simulink model "Sem1DemoSmallANDTOU_COPY"  (R2023a)
settings: Solver=ode23t  StartTime=0.0  StopTime=10  RelTol=1e-3
libraries: simulink x15, dspswit3 x9, simulink_extras x7, spspowerguiLib x1
settings Model: PacingRate=4  Creator=jakob  LastModifiedBy=matty

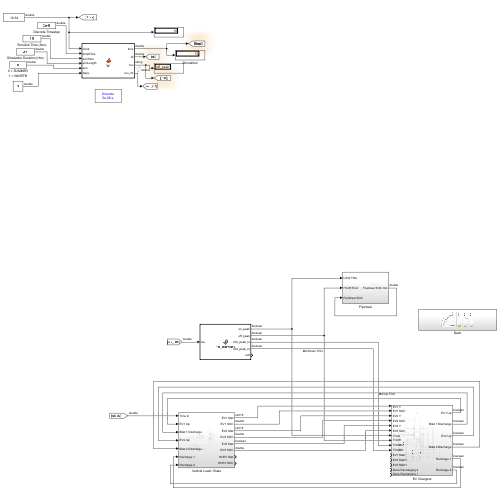
[thumbnail: Simulink's stored preview of the top-level diagram]
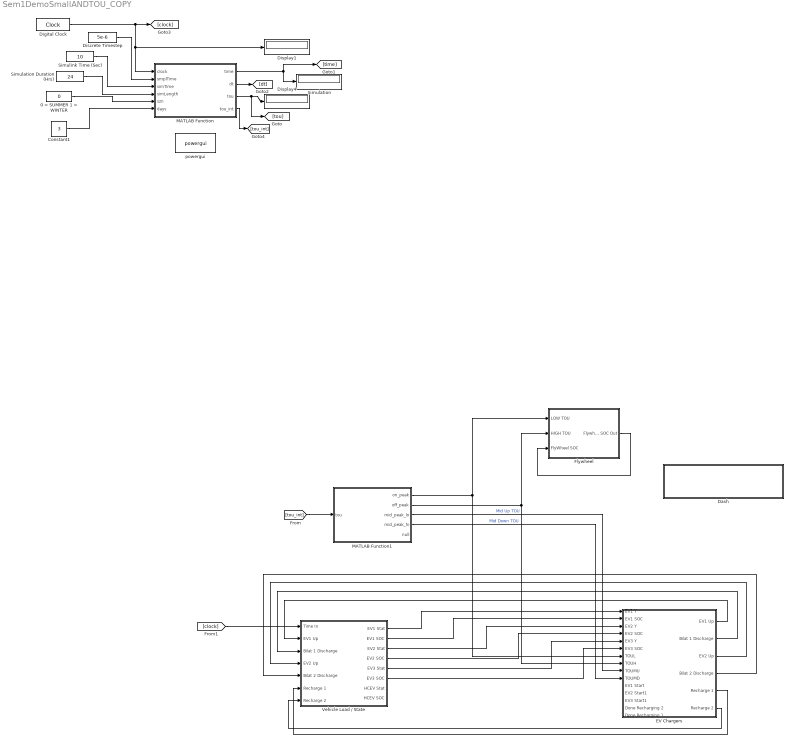
== system Sem1DemoSmallANDTOU_COPY ==
  0 = SUMMER 1 = WINTER : Constant  Value=0
  Constant1 : Constant  Value=3
  Dash : Subsystem
  Digital Clock : DigitalClock  SampleTime=5e-6
  Discrete Timestep : Constant  Value=5e-6
  Display1 : Display
  Display4 : Display
  EV Chargers : Subsystem
  Flywheel : Subsystem  StopFcn=CapTest
  MATLAB Function : MATLAB Function  TreatAsAtomicUnit=on
  MATLAB Function1 : MATLAB Function  TreatAsAtomicUnit=on
  Simulation : Display
  Simulation Duration (Hrs) : Constant  Value=24
  Simulink Time (Sec) : Constant  Value=10
  Vehicle Load / State : Subsystem
  powergui : spspowerguiLib/powergui  Priority=1  SimulationMode=Discrete  SampleTime=5e-6  frequency=60  Iterations=50  frequencyindice=0  Pbase=100e6  ErrMax=1e-4  UnitsV=kV  UnitsW=MW  buscounter=0  FunctionMessages=off  echomessages=off  EnableUseOfTLC=off  CurrentSourceSwitches=off  DisableSnubberDevices=off  DisableRonSwitches=off  DisableVfSwitches=off  DisplayEquations=off  AutomaticDiscreteSolvers=off  SolverType=Tustin/Backward Euler (TBE)  Interpol=off  ExternalGateDelay=off  methode=off  Ts=100  x0status=blocks  SPID=on  SwTol=0  HookPort=off  NonlinearTolerance=1e-4  nMaxIteration=100  ContinueOnMaxIteration=off  RestoreLinks=warning  ResistiveCurrentMeasurement=off  Frange=[0:2:500]  Ylog=off  Xlog=on  ShowGrid=off  save=off  variable=ZData  structure=0  ZoomFFT=off  StartTime=0.0  cycles=1  DisplayStyle=1  fundamental=60  FreqAxis=off  MaxFrequency=1000  frequencyindicesteady=1  RmsSteady=1  display=off
  wires:
  MATLAB Function1/1(on_peak) -> EV Chargers/7(TOUL), Flywheel/1(LOW TOU)
  Vehicle Load / State/1(EV1 Stat) -> EV Chargers/1(EV1 Y)
  Vehicle Load / State/2(EV1 SOC) -> EV Chargers/2(EV1 SOC)
  Vehicle Load / State/3(EV2 Stat) -> EV Chargers/3(EV2 Y)
  Vehicle Load / State/4(EV2 SOC) -> EV Chargers/4(EV2 SOC)
  Vehicle Load / State/5(EV3 Stat) -> EV Chargers/5(EV3 Y)
  Vehicle Load / State/6(EV3 SOC) -> EV Chargers/6(EV3 SOC)
  MATLAB Function1/2(off_peak) -> EV Chargers/8(TOUH), Flywheel/2(HIGH TOU)
  MATLAB Function1/3(mid_peak_lo) -> EV Chargers/9(TOUMU)  "Mid Up TOU"
  MATLAB Function1/4(mid_peak_hi) -> EV Chargers/10(TOUMD)  "Mid Down TOU"
  Flywheel/1(Flywheel SOC Out) -> Flywheel/3(FlyWheel SOC)
  EV Chargers/1(EV1 Up) -> Vehicle Load / State/2(EV1 Up)
  EV Chargers/2(Bilat 1 Discharge) -> Vehicle Load / State/3(Bilat 1 Discharge)
  EV Chargers/3(EV2 Up) -> Vehicle Load / State/4(EV2 Up)
  EV Chargers/4(Bilat 2 Discharge) -> Vehicle Load / State/5(Bilat 2 Discharge)
  EV Chargers/5(Recharge 1) -> Vehicle Load / State/6(Recharge 1)
  EV Chargers/6(Recharge 2) -> Vehicle Load / State/7(Recharge 2)
  MATLAB Function/4(tou_int) -> [tou_int]
  0 = SUMMER 1 = WINTER/1 -> MATLAB Function/5(szn)
  Constant1/1 -> MATLAB Function/6(days)
  MATLAB Function/2(dt) -> [dt]
  Simulink Time (Sec)/1 -> MATLAB Function/3(simTime)
  MATLAB Function/3(tou) -> [tou], Display4/1
  Discrete Timestep/1 -> MATLAB Function/2(smplTime)
  Digital Clock/1 -> [clock], MATLAB Function/1(clock), Display1/1
  MATLAB Function/1(time) -> [time], Simulation/1
  Simulation Duration (Hrs)/1 -> MATLAB Function/4(simLength)
  [tou_int] -> MATLAB Function1/1(tou)
  [clock] -> Vehicle Load / State/1(Time In)

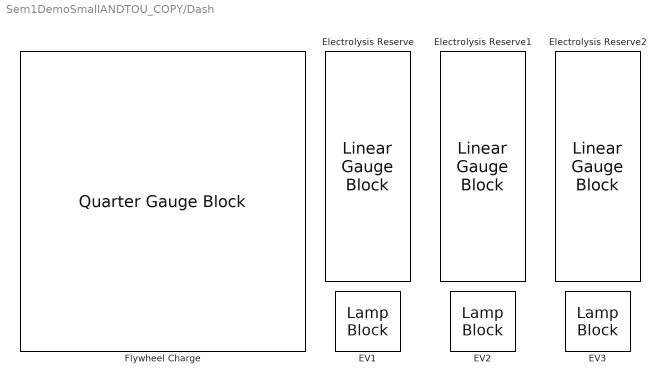
== system Sem1DemoSmallANDTOU_COPY/Dash ==
  EV1 : LampBlock  LabelPosition=Hide
  EV2 : LampBlock  LabelPosition=Hide
  EV3 : LampBlock  LabelPosition=Hide
  Electrolysis Reserve : LinearGaugeBlock  Tag=Flywheel %
  Electrolysis Reserve1 : LinearGaugeBlock  Tag=Flywheel %
  Electrolysis Reserve2 : LinearGaugeBlock  Tag=Flywheel %
  Flywheel Charge : QuarterGaugeBlock

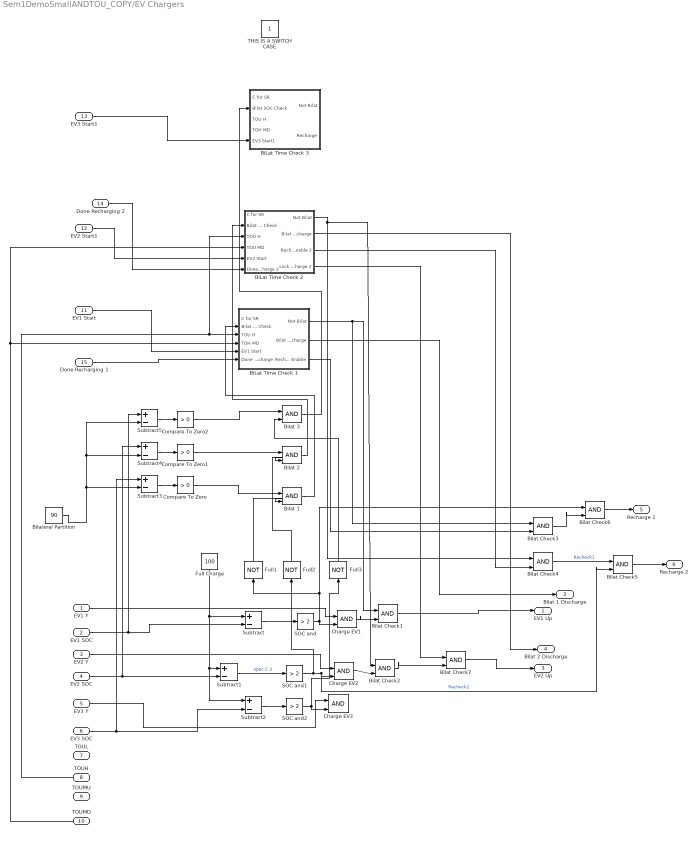
== system Sem1DemoSmallANDTOU_COPY/EV Chargers ==
  EV1 Y : Inport
  EV1 SOC : Inport  Port=2
  EV2 Y : Inport  Port=3
  EV2 SOC : Inport  Port=4
  EV3 Y : Inport  Port=5
  EV3 SOC : Inport  Port=6
  TOUL : Inport  Port=7
  TOUH : Inport  Port=8
  TOUMU : Inport  Port=9
  TOUMD : Inport  Port=10
  EV1 Start : Inport  Port=11
  EV2 Start1 : Inport  Port=12
  EV3 Start1 : Inport  Port=13
  Done Recharging 2 : Inport  Port=14
  Done Recharging 1 : Inport  Port=15
  BiLat Time Check 1 : Subsystem
  BiLat Time Check 2 : Subsystem
  BiLat Time Check 3 : Subsystem
  Bilat 1 : Logic  IconShape=distinctive  AllPortsSameDT=off  OutDataTypeStr=boolean
  Bilat 2 : Logic  IconShape=distinctive  AllPortsSameDT=off  OutDataTypeStr=boolean
  Bilat 3 : Logic  IconShape=distinctive  AllPortsSameDT=off  OutDataTypeStr=boolean
  Bilat Check{1..7} (7 alike) : Logic  IconShape=distinctive  AllPortsSameDT=off  OutDataTypeStr=boolean
  Bilateral Partition : Constant  Value=90
  Charge EV1 : Logic  IconShape=distinctive  AllPortsSameDT=off  OutDataTypeStr=boolean
  Charge EV2 : Logic  IconShape=distinctive  AllPortsSameDT=off  OutDataTypeStr=boolean
  Charge EV3 : Logic  IconShape=distinctive  AllPortsSameDT=off  OutDataTypeStr=boolean
  Compare To Zero : simulink/Logic and Bit Operations/Compare To Zero  relop=>  OutDataTypeStr=boolean
  Compare To Zero1 : simulink/Logic and Bit Operations/Compare To Zero  relop=>  OutDataTypeStr=boolean
  Compare To Zero2 : simulink/Logic and Bit Operations/Compare To Zero  relop=>  OutDataTypeStr=boolean
  Full Charge : Constant  Value=100
  Full1 : Logic  Operator=NOT  IconShape=distinctive  AllPortsSameDT=off  OutDataTypeStr=boolean
  Full2 : Logic  Operator=NOT  IconShape=distinctive  AllPortsSameDT=off  OutDataTypeStr=boolean
  Full3 : Logic  Operator=NOT  IconShape=distinctive  AllPortsSameDT=off  OutDataTypeStr=boolean
  SOC and : simulink/Logic and Bit Operations/Compare To Constant  relop=>  const=2  OutDataTypeStr=boolean
  SOC and1 : simulink/Logic and Bit Operations/Compare To Constant  relop=>  const=2  OutDataTypeStr=boolean
  SOC and2 : simulink/Logic and Bit Operations/Compare To Constant  relop=>  const=2  OutDataTypeStr=boolean
  Subtract{,1..5} (6 alike) : Sum  Inputs=+-
  THIS IS A SWITCH CASE : Constant
  EV1 Up : Outport
  Bilat 1 Discharge : Outport  Port=2
  EV2 Up : Outport  Port=3
  Bilat 2 Discharge : Outport  Port=4
  Recharge 1 : Outport  Port=5
  Recharge 2 : Outport  Port=6
  wires:
  Full Charge/1 -> Subtract2/1, Subtract1/1, Subtract/1
  EV1 SOC/1 -> Subtract5/1, Subtract/2
  EV2 Y/1 -> Charge EV2/1
  SOC and1/1 -> Bilat Check5/2, Charge EV2/2, Full2/1  "Recheck2"
  Subtract1/1 -> SOC and1/1  "Spec C 3"
  SOC and2/1 -> Full3/1, Charge EV3/2
  SOC and/1 -> Bilat Check6/1, Full1/1, Charge EV1/2
  Subtract/1 -> SOC and/1
  Subtract2/1 -> SOC and2/1
  EV3 SOC/1 -> Subtract3/1, Subtract2/2
  Charge EV2/1 -> Bilat Check2/2
  EV1 Y/1 -> Charge EV1/1
  EV3 Y/1 -> Charge EV3/1
  EV2 SOC/1 -> Subtract4/1, Subtract1/2
  Subtract3/1 -> Compare To Zero/1
  Subtract4/1 -> Compare To Zero1/1
  Subtract5/1 -> Compare To Zero2/1
  Full1/1 -> Bilat 1/2
  Compare To Zero/1 -> Bilat 1/1
  Compare To Zero1/1 -> Bilat 2/1
  Compare To Zero2/1 -> Bilat 3/1
  Full2/1 -> Bilat 2/2
  Full3/1 -> Bilat 3/2
  Bilateral Partition/1 -> Subtract4/2, Subtract5/2, Subtract3/2
  Bilat 3/1 -> BiLat Time Check 3/2(Bilat SOC Check)
  Bilat 2/1 -> BiLat Time Check 2/2(Bilat SOC Check)
  EV1 Start/1 -> BiLat Time Check 1/5(EV1 Start)
  Bilat 1/1 -> BiLat Time Check 1/2(Bilat SOC Check)
  TOUH/1 -> BiLat Time Check 2/3(TOU H), BiLat Time Check 1/3(TOU H)
  TOUMD/1 -> BiLat Time Check 2/4(TOU MD), BiLat Time Check 1/4(TOH MD)
  BiLat Time Check 1/2(Bilat Discharge) -> Bilat 1 Discharge/1
  BiLat Time Check 1/1(Not Bilat) -> Bilat Check3/1, Bilat Check1/1
  Charge EV1/1 -> Bilat Check1/2
  EV2 Start1/1 -> BiLat Time Check 2/5(EV2 Start)
  EV3 Start1/1 -> BiLat Time Check 3/5(EV3 Start1)
  BiLat Time Check 2/1(Not Bilat) -> Bilat Check4/1, Bilat Check2/1
  BiLat Time Check 2/2(Bilat Discharge) -> Bilat 2 Discharge/1
  Bilat Check2/1 -> Bilat Check7/2
  Bilat Check1/1 -> EV1 Up/1
  BiLat Time Check 1/3(Recharge Enable) -> Bilat Check3/2
  BiLat Time Check 2/3(Recharge Enable 2) -> Bilat Check4/2
  Done Recharging 2/1 -> BiLat Time Check 2/6(Done Recharge 2)
  Done Recharging 1/1 -> BiLat Time Check 1/6(Done Recharge)
  Bilat Check3/1 -> Bilat Check6/2
  Bilat Check4/1 -> Bilat Check5/1  "Recheck1"
  Bilat Check5/1 -> Recharge 2/1
  Bilat Check6/1 -> Recharge 1/1
  Bilat Check7/1 -> EV2 Up/1
  BiLat Time Check 2/4(Lock Out Recharge 2) -> Bilat Check7/1

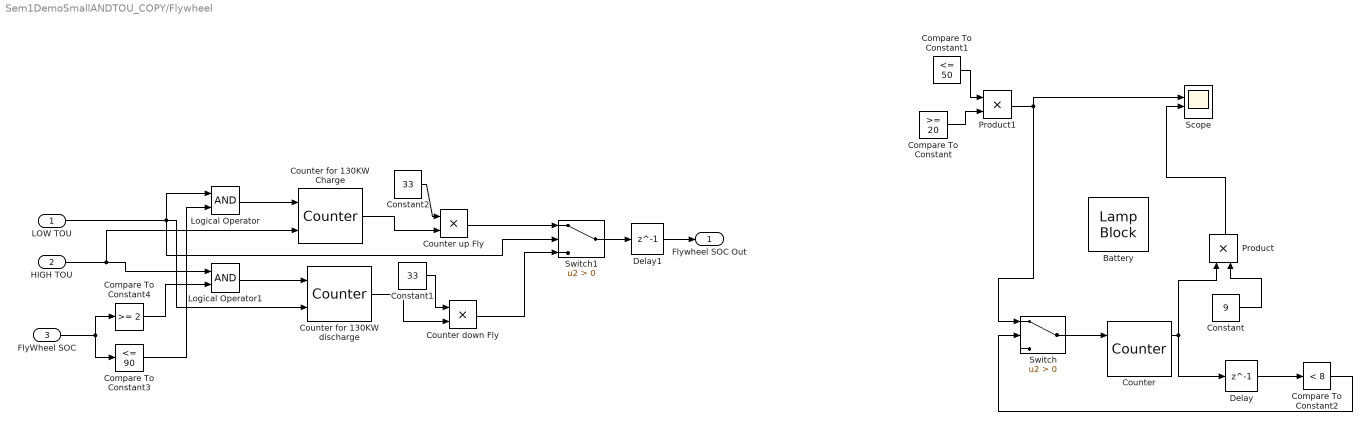
== system Sem1DemoSmallANDTOU_COPY/Flywheel ==
  LOW TOU : Inport
  HIGH TOU : Inport  Port=2
  FlyWheel SOC : Inport  Port=3
  Battery : LampBlock  LabelPosition=Hide  Icon=Battery
  Compare To Constant : simulink/Logic and Bit Operations/Compare To Constant  relop=>=  const=20  OutDataTypeStr=boolean
  Compare To Constant1 : simulink/Logic and Bit Operations/Compare To Constant  relop=<=  const=50  OutDataTypeStr=boolean
  Compare To Constant2 : simulink/Logic and Bit Operations/Compare To Constant  relop=<  const=8  OutDataTypeStr=boolean
  Compare To Constant3 : simulink/Logic and Bit Operations/Compare To Constant  relop=<=  const=90  OutDataTypeStr=boolean
  Compare To Constant4 : simulink/Logic and Bit Operations/Compare To Constant  relop=>=  const=2  OutDataTypeStr=boolean
  Constant : Constant  Value=9
  Constant1 : Constant  Value=33
  Constant2 : Constant  Value=33
  Counter : dspswit3/Counter  Direction=Up  CountEvent=Non-zero sample  CounterSize=User defined  MaxCount=100  InitialCount=0  Output=Count and Hit  HitValue=32  ResetInput=on  SamplesPerFrame=1  Ts=1  CntDtype=single  HitDtype=Logical
  Counter down Fly : Product
  Counter for 130KW Charge : dspswit3/Counter  Direction=Up  CountEvent=Non-zero sample  CounterSize=User defined  MaxCount=3  InitialCount=0  Output=Count  HitValue=32  ResetInput=on  SamplesPerFrame=1  Ts=1  CntDtype=single  HitDtype=Logical
  Counter for 130KW discharge : dspswit3/Counter  Direction=Down  CountEvent=Non-zero sample  CounterSize=User defined  MaxCount=10  InitialCount=3  Output=Count  HitValue=32  ResetInput=on  SamplesPerFrame=1  Ts=1  CntDtype=single  HitDtype=Logical
  Counter up Fly : Product
  Delay : Delay  DelayLength=1  InitialCondition=0
  Delay1 : Delay  DelayLength=1  InitialCondition=0
  Logical Operator : Logic  AllPortsSameDT=off  OutDataTypeStr=boolean
  Logical Operator1 : Logic  AllPortsSameDT=off  OutDataTypeStr=boolean
  Product : Product
  Product1 : Product
  Scope : Scope  NumInputPorts=4
  Switch : Switch  Criteria=u2 > Threshold  SaturateOnIntegerOverflow=off  InputSameDT=off
  Switch1 : Switch  Criteria=u2 > Threshold  SaturateOnIntegerOverflow=off  InputSameDT=off
  Flywheel SOC Out : Outport
  wires:
  Compare To Constant1/1 -> Product1/1
  Compare To Constant/1 -> Product1/2
  Counter/1 -> Product/1, Delay/1
  Product1/1 -> Switch/1, Scope/2
  Switch/1 -> Counter/1
  Compare To Constant2/1 -> Switch/2
  Delay/1 -> Compare To Constant2/1
  Constant/1 -> Product/2
  Product/1 -> Scope/3
  LOW TOU/1 -> Counter for 130KW discharge/2, Logical Operator/1, Switch1/2
  FlyWheel SOC/1 -> Compare To Constant4/1, Compare To Constant3/1
  Compare To Constant3/1 -> Logical Operator/2
  Compare To Constant4/1 -> Logical Operator1/2
  HIGH TOU/1 -> Counter for 130KW Charge/2, Logical Operator1/1
  Logical Operator1/1 -> Counter for 130KW discharge/1
  Constant1/1 -> Counter down Fly/1
  Counter for 130KW discharge/1 -> Counter down Fly/2
  Counter down Fly/1 -> Switch1/3
  Constant2/1 -> Counter up Fly/1
  Counter for 130KW Charge/1 -> Counter up Fly/2
  Logical Operator/1 -> Counter for 130KW Charge/1
  Counter up Fly/1 -> Switch1/1
  Switch1/1 -> Delay1/1
  Delay1/1 -> Flywheel SOC Out/1

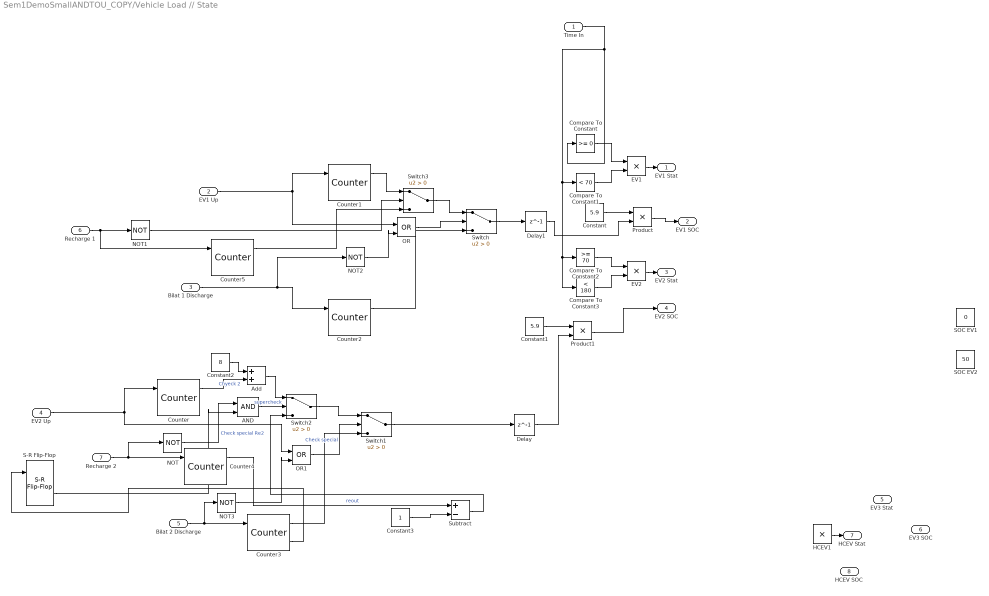
== system Sem1DemoSmallANDTOU_COPY/Vehicle Load // State ==
  Time In : Inport
  EV1 Up : Inport  Port=2
  Bilat 1 Discharge : Inport  Port=3
  EV2 Up : Inport  Port=4
  Bilat 2 Discharge : Inport  Port=5
  Recharge 1 : Inport  Port=6
  Recharge 2 : Inport  Port=7
  AND : Logic  IconShape=distinctive  AllPortsSameDT=off  OutDataTypeStr=boolean
  Add : Sum
  Compare To Constant : simulink/Logic and Bit Operations/Compare To Constant  relop=>=  const=0  OutDataTypeStr=boolean
  Compare To Constant1 : simulink/Logic and Bit Operations/Compare To Constant  relop=<  const=70  OutDataTypeStr=boolean
  Compare To Constant2 : simulink/Logic and Bit Operations/Compare To Constant  relop=>=  const=70  OutDataTypeStr=boolean
  Compare To Constant3 : simulink/Logic and Bit Operations/Compare To Constant  relop=<  const=180  OutDataTypeStr=boolean
  Constant : Constant  Value=5.9
  Constant1 : Constant  Value=5.9
  Constant2 : Constant  Value=8
  Constant3 : Constant
  Counter : dspswit3/Counter  Direction=Up  CountEvent=Non-zero sample  CounterSize=User defined  MaxCount=17  InitialCount=0  Output=Count and Hit  HitValue=9  ResetInput=on  SamplesPerFrame=1  Ts=1  CntDtype=single  HitDtype=Logical
  Counter1 : dspswit3/Counter  Direction=Up  CountEvent=Non-zero sample  CounterSize=User defined  MaxCount=100  InitialCount=0  Output=Count and Hit  HitValue=32  ResetInput=on  SamplesPerFrame=1  Ts=1  CntDtype=single  HitDtype=Logical
  Counter2 : dspswit3/Counter  Direction=Down  CountEvent=Non-zero sample  CounterSize=User defined  MaxCount=100  InitialCount=17  Output=Count and Hit  HitValue=32  ResetInput=on  SamplesPerFrame=1  Ts=1  CntDtype=single  HitDtype=Logical
  Counter3 : dspswit3/Counter  Direction=Down  CountEvent=Non-zero sample  CounterSize=User defined  MaxCount=17  InitialCount=17  Output=Count and Hit  HitValue=15  ResetInput=on  SamplesPerFrame=1  Ts=1  CntDtype=single  HitDtype=Logical
  Counter4 : dspswit3/Counter  Direction=Up  CountEvent=Non-zero sample  CounterSize=User defined  MaxCount=18  InitialCount=15  Output=Count and Hit  HitValue=100  ResetInput=on  SamplesPerFrame=1  Ts=1  CntDtype=single  HitDtype=Logical
  Counter5 : dspswit3/Counter  Direction=Up  CountEvent=Non-zero sample  CounterSize=User defined  MaxCount=100  InitialCount=15  Output=Count and Hit  HitValue=32  ResetInput=on  SamplesPerFrame=1  Ts=1  CntDtype=single  HitDtype=Logical
  Delay : Delay  DelayLength=1  InitialCondition=0
  Delay1 : Delay  DelayLength=1  InitialCondition=0
  EV1 : Product
  EV2 : Product
  HCEV1 : Product
  NOT{,1..3} (4 alike) : Logic  Operator=NOT  IconShape=distinctive  AllPortsSameDT=off  OutDataTypeStr=boolean
  OR : Logic  Operator=OR  IconShape=distinctive  AllPortsSameDT=off  OutDataTypeStr=boolean
  OR1 : Logic  Operator=OR  IconShape=distinctive  AllPortsSameDT=off  OutDataTypeStr=boolean
  Product : Product
  Product1 : Product
  S-R Flip-Flop : simulink_extras/Flip Flops/S-R Flip-Flop  initial_condition=0
  SOC EV1 : Constant  Value=0
  SOC EV2 : Constant  Value=50
  Subtract : Sum  Inputs=+-
  Switch{,1..3} (4 alike) : Switch  Criteria=u2 > Threshold  SaturateOnIntegerOverflow=off  InputSameDT=off
  EV1 Stat : Outport
  EV1 SOC : Outport  Port=2
  EV2 Stat : Outport  Port=3
  EV2 SOC : Outport  Port=4
  EV3 Stat : Outport  Port=5
  EV3 SOC : Outport  Port=6
  HCEV Stat : Outport  Port=7
  HCEV SOC : Outport  Port=8
  wires:
  Time In/1 -> Compare To Constant3/1, Compare To Constant2/1, Compare To Constant1/1, Compare To Constant/1
  Compare To Constant3/1 -> EV2/2
  Compare To Constant2/1 -> EV2/1
  Compare To Constant/1 -> EV1/1
  Compare To Constant1/1 -> EV1/2
  EV2/1 -> EV2 Stat/1
  HCEV1/1 -> HCEV Stat/1
  EV1/1 -> EV1 Stat/1
  EV2 Up/1 -> OR1/1, Counter/1
  EV1 Up/1 -> OR/1, Counter1/1
  Bilat 1 Discharge/1 -> NOT2/1, Counter2/1
  Switch/1 -> Delay1/1
  Counter2/1 -> Switch/3
  Switch1/1 -> Delay/1
  Bilat 2 Discharge/1 -> NOT3/1, Counter3/1
  Switch2/1 -> Switch1/1
  Counter/1 -> Add/2  "Chyeck 2"
  Recharge 2/1 -> NOT/1, Counter4/1
  NOT/1 -> AND/1  "Check special Re2"
  Counter5/1 -> Switch3/3
  Recharge 1/1 -> Counter5/1, NOT1/1
  Counter1/1 -> Switch3/1
  Switch3/1 -> Switch/1
  NOT1/1 -> Switch3/2
  Delay/1 -> Product1/2
  Delay1/1 -> Product/2
  Constant/1 -> Product/1
  Product/1 -> EV1 SOC/1
  OR/1 -> Switch/2
  NOT2/1 -> OR/2
  NOT3/1 -> OR1/2
  OR1/1 -> Switch1/2  "Check special"
  Constant1/1 -> Product1/1
  Product1/1 -> EV2 SOC/1
  Constant2/1 -> Add/1
  Add/1 -> Switch2/1
  Counter3/2 -> S-R Flip-Flop/1
  S-R Flip-Flop/2 -> AND/2
  AND/1 -> Switch2/2  "supercheck"
  Counter3/1 -> Switch1/3
  Counter4/1 -> Subtract/1  "reout"
  Constant3/1 -> Subtract/2
  Subtract/1 -> Switch2/3

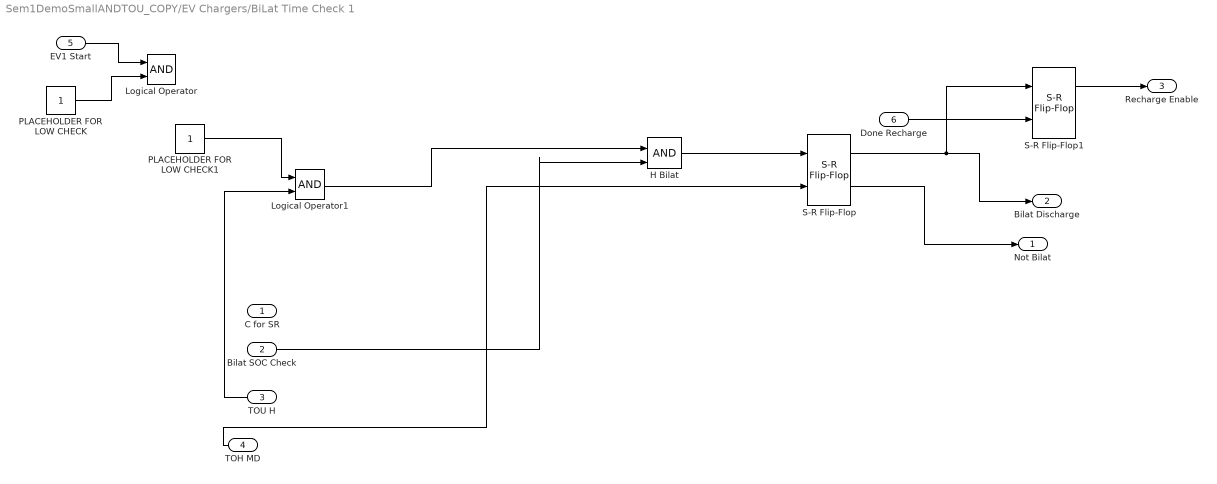
== system Sem1DemoSmallANDTOU_COPY/EV Chargers/BiLat Time Check 1 ==
  C for SR : Inport
  Bilat SOC Check : Inport  Port=2
  TOU H : Inport  Port=3
  TOH MD : Inport  Port=4
  EV1 Start : Inport  Port=5
  Done Recharge : Inport  Port=6
  H Bilat : Logic  IconShape=distinctive  AllPortsSameDT=off  OutDataTypeStr=boolean
  Logical Operator : Logic  AllPortsSameDT=off  OutDataTypeStr=boolean
  Logical Operator1 : Logic  AllPortsSameDT=off  OutDataTypeStr=boolean
  PLACEHOLDER FOR LOW CHECK : Constant
  PLACEHOLDER FOR LOW CHECK1 : Constant
  S-R Flip-Flop : simulink_extras/Flip Flops/S-R Flip-Flop  initial_condition=0
  S-R Flip-Flop1 : simulink_extras/Flip Flops/S-R Flip-Flop  initial_condition=0
  Not Bilat : Outport
  Bilat Discharge : Outport  Port=2
  Recharge Enable : Outport  Port=3
  wires:
  TOH MD/1 -> S-R Flip-Flop/2
  Logical Operator1/1 -> H Bilat/1
  PLACEHOLDER FOR LOW CHECK1/1 -> Logical Operator1/1
  H Bilat/1 -> S-R Flip-Flop/1
  S-R Flip-Flop/1 -> S-R Flip-Flop1/1, Bilat Discharge/1
  S-R Flip-Flop/2 -> Not Bilat/1
  Bilat SOC Check/1 -> H Bilat/2
  TOU H/1 -> Logical Operator1/2
  PLACEHOLDER FOR LOW CHECK/1 -> Logical Operator/2
  EV1 Start/1 -> Logical Operator/1
  S-R Flip-Flop1/1 -> Recharge Enable/1
  Done Recharge/1 -> S-R Flip-Flop1/2

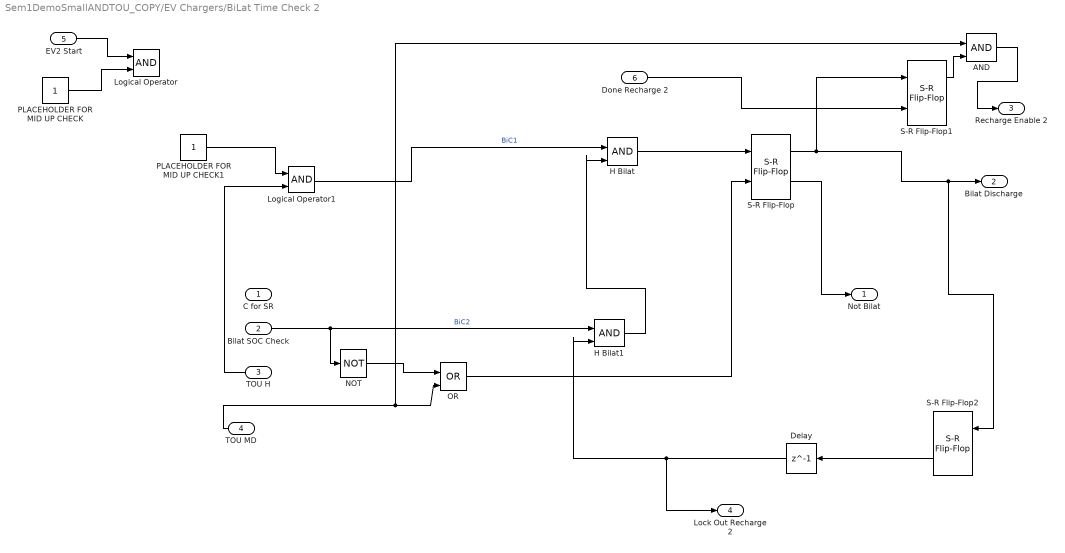
== system Sem1DemoSmallANDTOU_COPY/EV Chargers/BiLat Time Check 2 ==
  C for SR : Inport
  Bilat SOC Check : Inport  Port=2
  TOU H : Inport  Port=3
  TOU MD : Inport  Port=4
  EV2 Start : Inport  Port=5
  Done Recharge 2 : Inport  Port=6
  AND : Logic  IconShape=distinctive  AllPortsSameDT=off  OutDataTypeStr=boolean
  Delay : Delay  DelayLength=1  InitialCondition=0
  H Bilat : Logic  IconShape=distinctive  AllPortsSameDT=off  OutDataTypeStr=boolean
  H Bilat1 : Logic  IconShape=distinctive  AllPortsSameDT=off  OutDataTypeStr=boolean
  Logical Operator : Logic  AllPortsSameDT=off  OutDataTypeStr=boolean
  Logical Operator1 : Logic  AllPortsSameDT=off  OutDataTypeStr=boolean
  NOT : Logic  Operator=NOT  IconShape=distinctive  AllPortsSameDT=off  OutDataTypeStr=boolean
  OR : Logic  Operator=OR  IconShape=distinctive  AllPortsSameDT=off  OutDataTypeStr=boolean
  PLACEHOLDER FOR MID UP CHECK : Constant
  PLACEHOLDER FOR MID UP CHECK1 : Constant
  S-R Flip-Flop : simulink_extras/Flip Flops/S-R Flip-Flop  initial_condition=0
  S-R Flip-Flop1 : simulink_extras/Flip Flops/S-R Flip-Flop  initial_condition=0
  S-R Flip-Flop2 : simulink_extras/Flip Flops/S-R Flip-Flop  initial_condition=0
  Not Bilat : Outport
  Bilat Discharge : Outport  Port=2
  Recharge Enable 2 : Outport  Port=3
  Lock Out Recharge 2 : Outport  Port=4
  wires:
  Logical Operator1/1 -> H Bilat/1  "BiC1"
  PLACEHOLDER FOR MID UP CHECK1/1 -> Logical Operator1/1
  S-R Flip-Flop/1 -> S-R Flip-Flop1/1, S-R Flip-Flop2/1, Bilat Discharge/1
  H Bilat/1 -> S-R Flip-Flop/1
  S-R Flip-Flop/2 -> Not Bilat/1
  Bilat SOC Check/1 -> H Bilat1/1, NOT/1  "BiC2"
  TOU H/1 -> Logical Operator1/2
  EV2 Start/1 -> Logical Operator/1
  PLACEHOLDER FOR MID UP CHECK/1 -> Logical Operator/2
  TOU MD/1 -> AND/1, OR/2
  Done Recharge 2/1 -> S-R Flip-Flop1/2
  AND/1 -> Recharge Enable 2/1
  OR/1 -> S-R Flip-Flop/2
  NOT/1 -> OR/1
  H Bilat1/1 -> H Bilat/2
  S-R Flip-Flop2/2 -> Delay/1
  Delay/1 -> Lock Out Recharge 2/1, H Bilat1/2
  S-R Flip-Flop1/1 -> AND/2

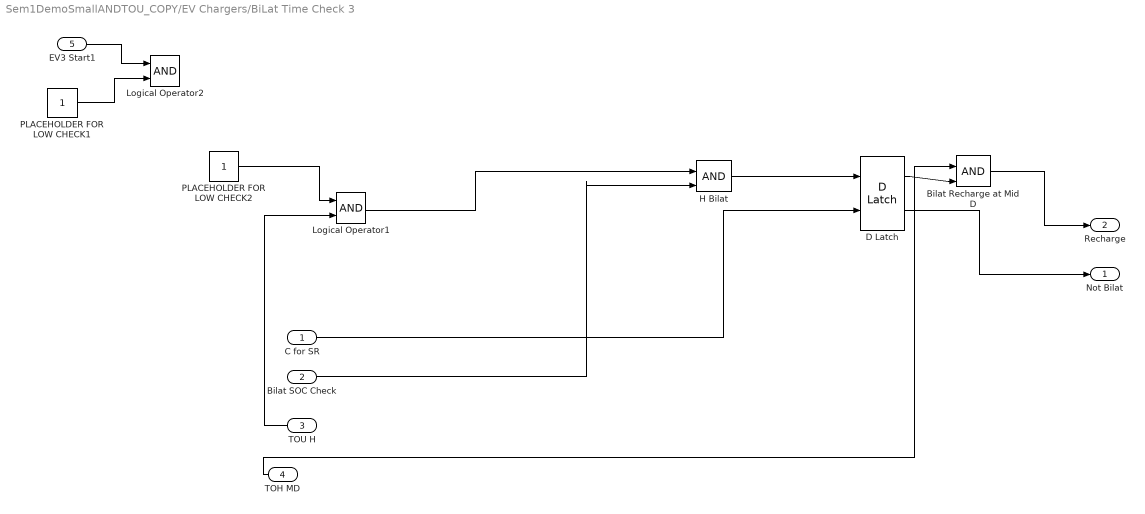
== system Sem1DemoSmallANDTOU_COPY/EV Chargers/BiLat Time Check 3 ==
  C for SR : Inport
  Bilat SOC Check : Inport  Port=2
  TOU H : Inport  Port=3
  TOH MD : Inport  Port=4
  EV3 Start1 : Inport  Port=5
  Bilat Recharge at Mid D : Logic  IconShape=distinctive  AllPortsSameDT=off  OutDataTypeStr=boolean
  D Latch : simulink_extras/Flip Flops/D Latch
  H Bilat : Logic  IconShape=distinctive  AllPortsSameDT=off  OutDataTypeStr=boolean
  Logical Operator1 : Logic  AllPortsSameDT=off  OutDataTypeStr=boolean
  Logical Operator2 : Logic  AllPortsSameDT=off  OutDataTypeStr=boolean
  PLACEHOLDER FOR LOW CHECK1 : Constant
  PLACEHOLDER FOR LOW CHECK2 : Constant
  Not Bilat : Outport
  Recharge : Outport  Port=2
  wires:
  TOH MD/1 -> Bilat Recharge at Mid D/1
  Logical Operator1/1 -> H Bilat/1
  PLACEHOLDER FOR LOW CHECK2/1 -> Logical Operator1/1
  Bilat Recharge at Mid D/1 -> Recharge/1
  H Bilat/1 -> D Latch/1
  D Latch/1 -> Bilat Recharge at Mid D/2
  D Latch/2 -> Not Bilat/1
  C for SR/1 -> D Latch/2
  Bilat SOC Check/1 -> H Bilat/2
  TOU H/1 -> Logical Operator1/2
  EV3 Start1/1 -> Logical Operator2/1
  PLACEHOLDER FOR LOW CHECK1/1 -> Logical Operator2/2

== matlab function Sem1DemoSmallANDTOU_COPY/MATLAB Function1 ==
  data: tou input; on_peak output; off_peak output; mid_peak_lo output; mid_peak_hi output; null output
function [on_peak, off_peak, mid_peak_lo, mid_peak_hi, null] = tou_translate(tou)

if tou == 0
    on_peak = false;
    off_peak = false;
    mid_peak_lo = false;
    mid_peak_hi = false;
    null = true;
elseif tou == 1
    on_peak = false;
    off_peak = true;
    mid_peak_lo = false;
    mid_peak_hi = false;
    null = false;
elseif tou == 2
    on_peak = false;
    off_peak = false;
    mid_peak_lo = true;
    mid_peak_hi = false;
    null = false;
elseif tou == 3
    on_peak = false;
    off_peak = false;
    mid_peak_lo = false;
    mid_peak_hi = true;
    null = false;
elseif tou == 4
    on_peak = true;
    off_peak = false;
    mid_peak_lo = false;
    mid_peak_hi = false;
    null = false;
else
    on_peak = false;
    off_peak = false;
    mid_peak_lo = false;
    mid_peak_hi = false;
    null = true;
end

end

== matlab function Sem1DemoSmallANDTOU_COPY/MATLAB Function ==
  data: clock input; time output; smplTime input; dt output; tou output; simTime input; simLength input; szn input; days input; tou_int output
function [time, dt, tou, tou_int] = fcn(clock, smplTime, simTime, simLength, szn, days)
    % Adjusted simulation time to span over 'days' days
    % First, calculate the total simulation time in hours for the given number of days
    totalSimHours = simLength * days;
    
    % Convert clock (in seconds) to actual simulation time (in hours)
    % Instead of scaling the entire simulation to fit within a single day,
    % scale it based on the total simulation hours specified by 'days'
    scalingFactor = totalSimHours / (simTime / 3600);
    scaledTime = clock / 3600 * scalingFactor; % Convert clock to hours and scale based on totalSimHours
    
    tou = "null";
    tou_int = 0;

    % Outputs
    time = scaledTime; % The scaled simulation time in hours, adjusted for multiple days
    dt = (smplTime / simTime) * scaledTime; % The timestep in hours

    % Determine the time of use (TOU) state based on the scaled simulation time
    % For TOU calculations, use mod(time, 24) to determine the time of day for TOU state decisions
    currentTimeOfDay = mod(time, 24);

    % Assuming the 'hrs' variable represents an hour in the context of currentTimeOfDay
    hrs = 1; % 1 hour in terms of scaled simulation time

    % Update TOU state checks to use currentTimeOfDay for daily cycle logic
    if szn == 0
        if (currentTimeOfDay >= 0*hrs && currentTimeOfDay <= 7*hrs) || (currentTimeOfDay > 19*hrs && currentTimeOfDay <= 24*hrs)
            tou = "off_peak";
            tou_int = 1; % off peak
        elseif (currentTimeOfDay > 7*hrs && currentTimeOfDay <= 11*hrs)
            tou = "mid_peak_hi";
            tou_int = 3; % mid peak hi
        elseif (currentTimeOfDay > 11*hrs && currentTimeOfDay <= 17*hrs)
            tou = "on_peak";
            tou_int = 4; % on peak
        elseif (currentTimeOfDay > 17*hrs && currentTimeOfDay <= 19*hrs)
            tou = "mid_peak_lo";
            tou_int = 2; % mid peak lo
        else
            tou = "null";
            tou_int = 0; % null/error
        end
    elseif szn == 1
        if (currentTimeOfDay >= 0*hrs && currentTimeOfDay <= 7*hrs) || (currentTimeOfDay > 19*hrs && currentTimeOfDay <= 24*hrs)
            tou = "off_peak";
            tou_int = 1; % off peak
        elseif (currentTimeOfDay > 7*hrs && currentTimeOfDay <= 11*hrs)
            tou = "on_peak";
            tou_int = 4; % on peak
        elseif (currentTimeOfDay > 11*hrs && currentTimeOfDay <= 17*hrs)
            tou = "mid_peak_lo";
            tou_int = 2; % mid peak lo
        elseif (currentTimeOfDay > 17*hrs && currentTimeOfDay <= 19*hrs)
            tou = "on_peak";
            tou_int = 4; % on peak
        else
            tou = "null";
        end
    end 
end
